simulink model "real_LAB3_EST"  (R2025b)
settings: Solver=ode3  StartTime=0.0  StopTime=10  FixedStep=0.001  RelTol=1e-3
values from neighbouring files (symbols this model uses):
  t0 = 0.2    [diScorta.m]    (also in real_LAB3.m; real_estimation.m)
  t1 = 0.7    [diScorta.m]    (also in real_LAB3.m; real_estimation.m)
  Ts = 0.001    [diScorta.m]    (also in real_LAB3.m; real_estimation.m; sim_LAB3.m)
undefined symbols (not defined in the file or in its folder): DiscIntNeverNeededParam, National_Instruments, PCI, sens
libraries: sldrtlib x1, simulink x1
settings Model: SimulationMode=external  ExtModeTrigDuration=100001  Creator=delpratogi  LastModifiedBy=Gioele
settings HardwareCC: ProdBitPerLong=64.0  ProdHWDeviceType=Intel->x86-64 (Linux 64)
settings RTWCC: SystemTargetFile=sldrt.tlc  TemplateMakefile=sldrt.tmf  RTWCompilerOptimization=on  Description=Simulink Desktop Real-Time
settings CodeAppCC: MaxIdLength=95.0
settings SimulinkDesktopRealTimeCC: ExtModeTransport=0.0  ExtModeStaticAllocSize=1000000.0  TargetLibSuffix=_sldrt.a  TargetPreCompLibLocation=C:\Program Files\MATLAB\R2025b\toolbox\sldrt\lib\win64  MultiwordLength=2048.0  DynamicStringBufferSize=256.0  ParMdlRefBuildCompliant=on  PreserveMATLABNamespacesInGeneratedCode=on  SubcomponentCodeInterfacePackaging=Reusable function

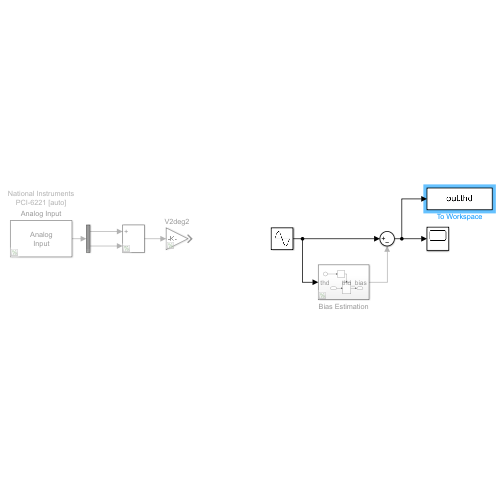
[thumbnail: Simulink's stored preview of the top-level diagram]
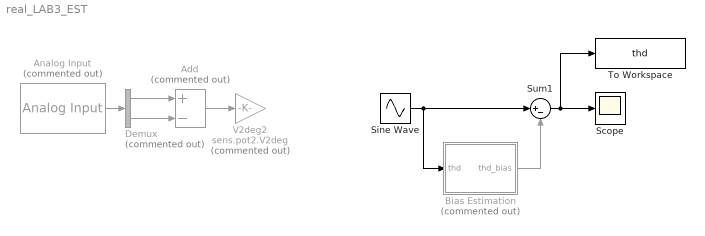
== system real_LAB3_EST ==
  Add : Sum  Commented=on  Inputs=+-
  Analog Input : sldrtlib/Analog Input  Commented=on  SampleTime=0.001  MaxMissedTicks=10  ShowMissedTicks=off  YieldWhenWaiting=off  DrvName=National_Instruments/PCI-6221  DrvAddress=4294967295  DrvOptions=[0 0 0 2 0]  Channels=[3,2]  RangeMode=1  VoltRange=2  DataType=1
      settings: AttributesFormatString=National Instruments\nPCI-6221 [auto]
  Bias Estimation : Subsystem  Commented=on
  Demux : Demux  Commented=on  Outputs=2
  Scope : Scope
      settings: ActiveDisplayYMinimum=-1  ActiveDisplayYMaximum=1
  Sine Wave : Sin  SampleTime=0
  Sum1 : Sum  Inputs=|+-
  To Workspace : ToWorkspace  VariableName=thd  SaveFormat=Structure With Time  SampleTime=Ts
  V2deg2 : Gain  Commented=on  Gain=sens.pot2.V2deg
  wires:
  Demux/1 -> Add/1
  Sine Wave/1 -> Bias Estimation/1(thd), Sum1/1
  Analog Input/1 -> Demux/1
  Add/1 -> V2deg2/1
  Sum1/1 -> Scope/1, To Workspace/1
  Bias Estimation/1(thd_bias) -> Sum1/2
  Demux/2 -> Add/2

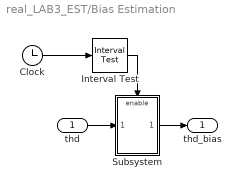
== system real_LAB3_EST/Bias Estimation ==
  thd : Inport
  Clock : Clock
  Interval Test : simulink/Logic and Bit Operations/Interval Test  IntervalClosedRight=on  uplimit=t1  IntervalClosedLeft=on  lowlimit=t0  OutDataTypeStr=boolean
  Subsystem : Subsystem
  thd_bias : Outport
  wires:
  Interval Test/1 -> Subsystem/Enable
  thd/1 -> Subsystem/1(In1)
  Subsystem/1(Out1) -> thd_bias/1
  Clock/1 -> Interval Test/1

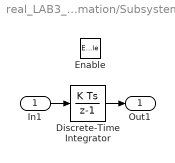
== system real_LAB3_EST/Bias Estimation/Subsystem ==
  In1 : Inport
  Enable : EnablePort
  Discrete-Time Integrator : DiscreteIntegrator  gainval=1/0.5  SampleTime=Ts  ICPrevOutput=DiscIntNeverNeededParam  ICPrevScaledInput=DiscIntNeverNeededParam
  Out1 : Outport
  wires:
  In1/1 -> Discrete-Time Integrator/1
  Discrete-Time Integrator/1 -> Out1/1
